simulink model "QuadrotorSim"  (R2019a)
settings: Solver=VariableStepAuto  StartTime=0.0  StopTime=inf  RelTol=1e-3
InitFcn:
  | close all; clear; clc;
  | mdl_quadrotor;
  | Para.d = 0.225;
  | Para.cT = 1.105e-5;
  | Para.cM = 1.779e-07;
  | Para.m = 1.4;
  | Para.Inertia = diag([0.0211, 0.0219, 0.0366]);
  | 
  | g = 9.8;
libraries: simulink x6, shared6dof x1, roblocks x1
settings Model: Creator=Administrator  LastModifiedBy=Cybaster
settings DataIOCC: ReturnWorkspaceOutputs=off
settings DebuggingCC: ArithmeticOperatorsInVariantConditions=warning

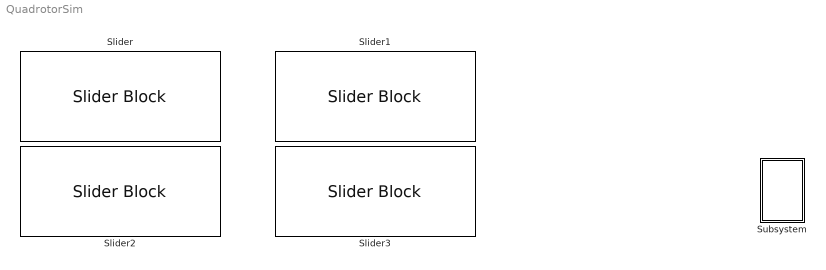
== system QuadrotorSim ==
  Slider : SliderBlock  ScaleMin=-2  ScaleMax=2
  Slider1 : SliderBlock  ScaleMin=-2  ScaleMax=2
  Slider2 : SliderBlock  ScaleMax=10
  Slider3 : SliderBlock  ScaleMin=-3.1400000000000001  ScaleMax=3.1400000000000001
  Subsystem : Subsystem

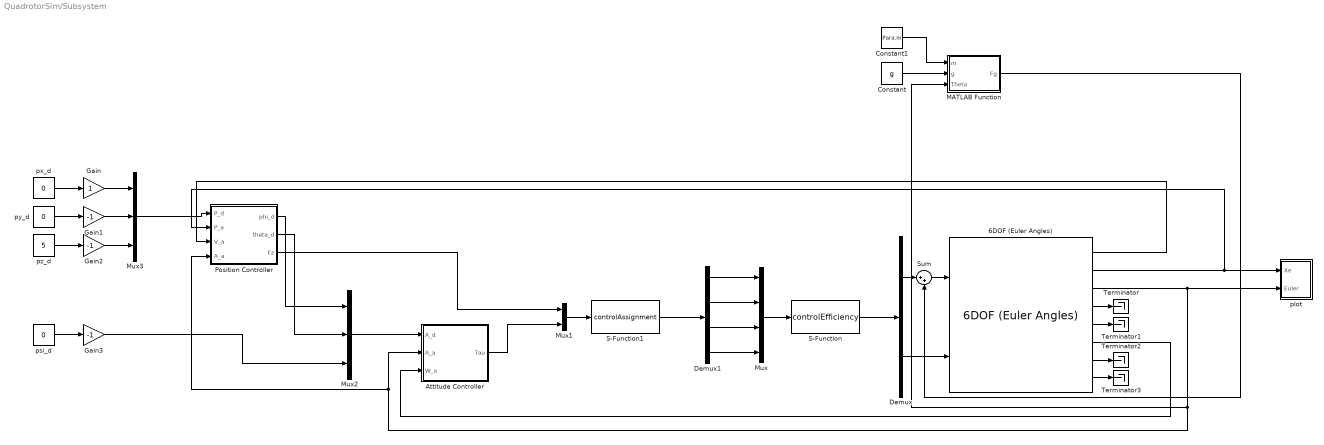
== system QuadrotorSim/Subsystem ==
  6DOF (Euler Angles) : shared6dof/6DOF (Euler Angles)  units=Metric (MKS)  mtype=Fixed  rep=Euler Angles  xme_0=[0.0 0.0 0.0]  Vm_0=[0.0 0.0 0.0]  eul_0=[0.0 0.0 0.0]  pm_0=[0.0 0.0 0.0]  mass_0=Para.m  mass_e=0.5  mass_f=2.0  inertia=Para.Inertia  inertia_e=eye(3)  inertia_f=2*eye(3)  k_quat=1.0  vre_flag=on  abi_flag=off  aMode=0  xme_statename=''  Vm_statename=''  eul_statename=''  quat_statename=''  pm_statename=''  mass_statename=''
      settings: SourceProductBaseCode=AE
  Attitude Controller : Subsystem
  Constant : Constant  Value=g
  Constant1 : Constant  Value=Para.m
  Demux : Demux  Outputs=2
  Demux1 : Demux
  Gain : Gain
  Gain1 : Gain  Gain=-1
  Gain2 : Gain  Gain=-1
  Gain3 : Gain  Gain=-1
  MATLAB Function : MATLAB Function  TreatAsAtomicUnit=on
  Mux : Mux
  Mux1 : Mux  Inputs=2
  Mux2 : Mux  Inputs=3
  Mux3 : Mux  Inputs=3
  Position Controller : Subsystem
  S-Function : S-Function  FunctionName=controlEfficiency  Parameters=Para  SFunctionDeploymentMode=off  EnableBusSupport=off
  S-Function1 : S-Function  FunctionName=controlAssignment  SFunctionDeploymentMode=off  EnableBusSupport=off
  Sum : Sum  Inputs=|++
  Terminator{,1..3} (4 alike) : Terminator
  plot : Subsystem
  psi_d : Constant  Value=0
  px_d : Constant  Value=0
  py_d : Constant  Value=0
  pz_d : Constant  Value=5
  wires:
  Demux1/1 -> Mux/1
  Demux/2 -> 6DOF (Euler Angles)/2
  Position Controller/2(theta_d) -> Mux2/2
  Mux1/1 -> S-Function1/1
  Mux3/1 -> Position Controller/1(P_d)
  6DOF (Euler Angles)/7 -> Terminator2/1
  Demux1/3 -> Mux/3
  Demux/1 -> Sum/1
  6DOF (Euler Angles)/3 -> MATLAB Function/3(Theta), Attitude Controller/2(A_a), Position Controller/4(A_a), plot/2(Euler)
  S-Function/1 -> Demux/1
  6DOF (Euler Angles)/8 -> Terminator3/1
  6DOF (Euler Angles)/4 -> Terminator/1
  6DOF (Euler Angles)/5 -> Terminator1/1
  6DOF (Euler Angles)/1 -> Position Controller/3(V_a)
  Gain2/1 -> Mux3/3
  Constant/1 -> MATLAB Function/2(g)
  Position Controller/1(phi_d) -> Mux2/1
  Gain1/1 -> Mux3/2
  Demux1/4 -> Mux/4
  6DOF (Euler Angles)/2 -> Position Controller/2(P_a), plot/1(Xe)
  Mux/1 -> S-Function/1
  Gain/1 -> Mux3/1
  py_d/1 -> Gain1/1
  Mux2/1 -> Attitude Controller/1(A_d)
  MATLAB Function/1(Fg) -> Sum/2
  px_d/1 -> Gain/1
  Attitude Controller/1(Tau) -> Mux1/2
  Position Controller/3(Fz) -> Mux1/1
  Sum/1 -> 6DOF (Euler Angles)/1
  Demux1/2 -> Mux/2
  6DOF (Euler Angles)/6 -> Attitude Controller/3(W_a)
  psi_d/1 -> Gain3/1
  S-Function1/1 -> Demux1/1
  Constant1/1 -> MATLAB Function/1(m)
  pz_d/1 -> Gain2/1
  Gain3/1 -> Mux2/3

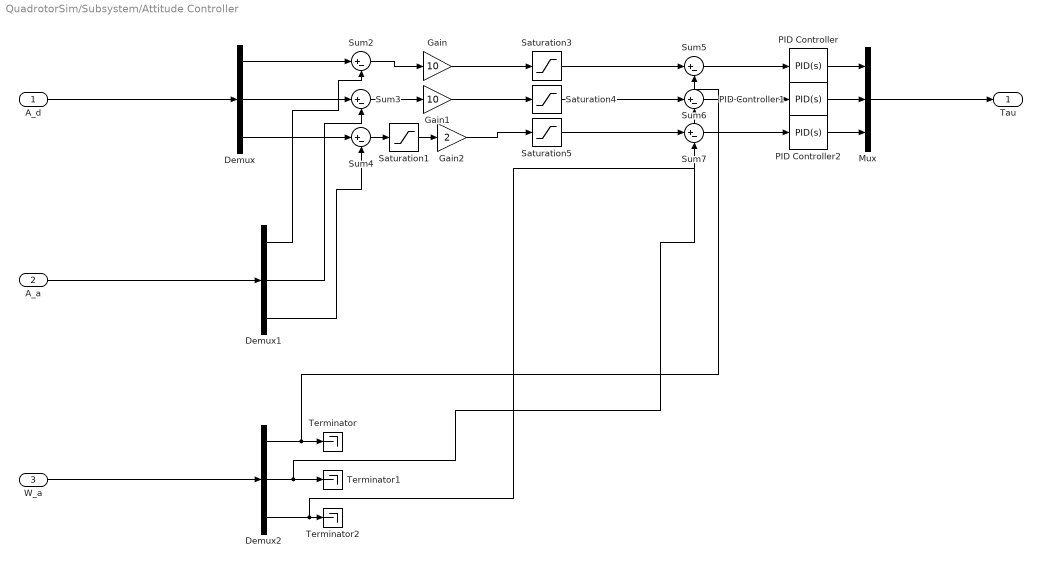
== system QuadrotorSim/Subsystem/Attitude Controller ==
  A_d : Inport
  A_a : Inport  Port=2
  W_a : Inport  Port=3
  Demux : Demux  Outputs=3
  Demux1 : Demux  Outputs=3
  Demux2 : Demux  Outputs=3
  Gain : Gain  Gain=10
  Gain1 : Gain  Gain=10
  Gain2 : Gain  Gain=2
  Mux : Mux  Inputs=3
  PID Controller : simulink/Continuous/PID Controller  Controller=PID  Form=Parallel  TimeDomain=Continuous-time  SampleTime=-1  IntegratorMethod=Forward Euler  FilterMethod=Forward Euler  ControllerParametersSource=internal  P=872359.79769725  I=16686702.0600055  D=-1838.38000156362  UseFilter=on  N=172.044274974478  TunerSelectOption=Transfer Function Based (PID Tuner App)  InitialConditionSource=internal  InitialConditionForIntegrator=0  InitialConditionForFilter=0  DifferentiatorICPrevScaledInput=0  ExternalReset=none  TrackingMode=off  Kt=1  LimitOutput=off  UpperSaturationLimit=inf  LowerSaturationLimit=-inf  LinearizeAsGain=on  AntiWindupMode=none  Kb=1  POutMin=[]  POutMax=[]  IOutMin=[]  IOutMax=[]  DOutMin=[]  DOutMax=[]  NOutMin=[]  NOutMax=[]  SumOutMin=[]  SumOutMax=[]  SaturationOutMin=[]  SaturationOutMax=[]  PParamMin=[]  PParamMax=[]  IParamMin=[]  IParamMax=[]  DParamMin=[]  DParamMax=[]  NParamMin=[]  NParamMax=[]  KbParamMin=[]  KbParamMax=[]  KtParamMin=[]  KtParamMax=[]  KbOutMin=[]  KbOutMax=[]  KtOutMin=[]  KtOutMax=[]  IntegratorOutMin=[]  IntegratorOutMax=[]  FilterOutMin=[]  FilterOutMax=[]  SumI1OutMin=[]  SumI1OutMax=[]  SumI2OutMin=[]  SumI2OutMax=[]  SumI3OutMin=[]  SumI3OutMax=[]  SumI4OutMin=[]  SumI4OutMax=[]  SumDOutMin=[]  SumDOutMax=[]  DifferentiatorOutMin=[]  DifferentiatorOutMax=[]  FilterDiffOutCoefMin=[]  FilterDiffOutCoefMax=[]  ReciprocalOutMin=[]  ReciprocalOutMax=[]  SumDenOutMin=[]  SumDenOutMax=[]  SumNumOutMin=[]  SumNumOutMax=[]  DivideOutMin=[]  DivideOutMax=[]  IntegratorContinuousStateAttributes=''  IntegratorStateMustResolveToSignalObject=off  IntegratorRTWStateStorageClass=Auto  FilterContinuousStateAttributes=''  FilterStateMustResolveToSignalObject=off  FilterRTWStateStorageClass=Auto  ParallelPVariant=InternalParameters  IdealPVariant=Disabled  IVariant=InternalParameters  DVariant=InternalParameters  IntegratorVariant=Continuous  SatVariant=Disabled  AWVariant=Passthrough  PCopyVariant=Disabled  TRVariant=Disabled  FdbkBlocksVariant=Forward  IdealPFdbkVariant=Disabled  SatFdbkVariant=Disabled  DerivativeFilterVariant=ContFilter  NVariant=InternalParameters  NCopyVariant=Disabled  FilterICVariant=InternalICsFilter  IntegratorICVariant=InternalICs  ExternalResetVariant=Disabled  TRSumVariant=Passthrough  SumFdbkVariant=Disabled  SumVariant=Sum_PID
  PID Controller1 : simulink/Continuous/PID Controller  Controller=PID  Form=Parallel  TimeDomain=Continuous-time  SampleTime=-1  IntegratorMethod=Forward Euler  FilterMethod=Forward Euler  ControllerParametersSource=internal  P=905409.552147454  I=17318885.4860674  D=-1908.02787827485  UseFilter=on  N=172.044274974478  TunerSelectOption=Transfer Function Based (PID Tuner App)  InitialConditionSource=internal  InitialConditionForIntegrator=0  InitialConditionForFilter=0  DifferentiatorICPrevScaledInput=0  ExternalReset=none  TrackingMode=off  Kt=1  LimitOutput=off  UpperSaturationLimit=inf  LowerSaturationLimit=-inf  LinearizeAsGain=on  AntiWindupMode=none  Kb=1  POutMin=[]  POutMax=[]  IOutMin=[]  IOutMax=[]  DOutMin=[]  DOutMax=[]  NOutMin=[]  NOutMax=[]  SumOutMin=[]  SumOutMax=[]  SaturationOutMin=[]  SaturationOutMax=[]  PParamMin=[]  PParamMax=[]  IParamMin=[]  IParamMax=[]  DParamMin=[]  DParamMax=[]  NParamMin=[]  NParamMax=[]  KbParamMin=[]  KbParamMax=[]  KtParamMin=[]  KtParamMax=[]  KbOutMin=[]  KbOutMax=[]  KtOutMin=[]  KtOutMax=[]  IntegratorOutMin=[]  IntegratorOutMax=[]  FilterOutMin=[]  FilterOutMax=[]  SumI1OutMin=[]  SumI1OutMax=[]  SumI2OutMin=[]  SumI2OutMax=[]  SumI3OutMin=[]  SumI3OutMax=[]  SumI4OutMin=[]  SumI4OutMax=[]  SumDOutMin=[]  SumDOutMax=[]  DifferentiatorOutMin=[]  DifferentiatorOutMax=[]  FilterDiffOutCoefMin=[]  FilterDiffOutCoefMax=[]  ReciprocalOutMin=[]  ReciprocalOutMax=[]  SumDenOutMin=[]  SumDenOutMax=[]  SumNumOutMin=[]  SumNumOutMax=[]  DivideOutMin=[]  DivideOutMax=[]  IntegratorContinuousStateAttributes=''  IntegratorStateMustResolveToSignalObject=off  IntegratorRTWStateStorageClass=Auto  FilterContinuousStateAttributes=''  FilterStateMustResolveToSignalObject=off  FilterRTWStateStorageClass=Auto  ParallelPVariant=InternalParameters  IdealPVariant=Disabled  IVariant=InternalParameters  DVariant=InternalParameters  IntegratorVariant=Continuous  SatVariant=Disabled  AWVariant=Passthrough  PCopyVariant=Disabled  TRVariant=Disabled  FdbkBlocksVariant=Forward  IdealPFdbkVariant=Disabled  SatFdbkVariant=Disabled  DerivativeFilterVariant=ContFilter  NVariant=InternalParameters  NCopyVariant=Disabled  FilterICVariant=InternalICsFilter  IntegratorICVariant=InternalICs  ExternalResetVariant=Disabled  TRSumVariant=Passthrough  SumFdbkVariant=Disabled  SumVariant=Sum_PID
  PID Controller2 : simulink/Continuous/PID Controller  Controller=PID  Form=Parallel  TimeDomain=Continuous-time  SampleTime=-1  IntegratorMethod=Forward Euler  FilterMethod=Forward Euler  ControllerParametersSource=internal  P=21140502.8119185  I=404380477.817044  D=-44550.7435063145  UseFilter=on  N=172.044274974478  TunerSelectOption=Transfer Function Based (PID Tuner App)  InitialConditionSource=internal  InitialConditionForIntegrator=0  InitialConditionForFilter=0  DifferentiatorICPrevScaledInput=0  ExternalReset=none  TrackingMode=off  Kt=1  LimitOutput=off  UpperSaturationLimit=inf  LowerSaturationLimit=-inf  LinearizeAsGain=on  AntiWindupMode=none  Kb=1  POutMin=[]  POutMax=[]  IOutMin=[]  IOutMax=[]  DOutMin=[]  DOutMax=[]  NOutMin=[]  NOutMax=[]  SumOutMin=[]  SumOutMax=[]  SaturationOutMin=[]  SaturationOutMax=[]  PParamMin=[]  PParamMax=[]  IParamMin=[]  IParamMax=[]  DParamMin=[]  DParamMax=[]  NParamMin=[]  NParamMax=[]  KbParamMin=[]  KbParamMax=[]  KtParamMin=[]  KtParamMax=[]  KbOutMin=[]  KbOutMax=[]  KtOutMin=[]  KtOutMax=[]  IntegratorOutMin=[]  IntegratorOutMax=[]  FilterOutMin=[]  FilterOutMax=[]  SumI1OutMin=[]  SumI1OutMax=[]  SumI2OutMin=[]  SumI2OutMax=[]  SumI3OutMin=[]  SumI3OutMax=[]  SumI4OutMin=[]  SumI4OutMax=[]  SumDOutMin=[]  SumDOutMax=[]  DifferentiatorOutMin=[]  DifferentiatorOutMax=[]  FilterDiffOutCoefMin=[]  FilterDiffOutCoefMax=[]  ReciprocalOutMin=[]  ReciprocalOutMax=[]  SumDenOutMin=[]  SumDenOutMax=[]  SumNumOutMin=[]  SumNumOutMax=[]  DivideOutMin=[]  DivideOutMax=[]  IntegratorContinuousStateAttributes=''  IntegratorStateMustResolveToSignalObject=off  IntegratorRTWStateStorageClass=Auto  FilterContinuousStateAttributes=''  FilterStateMustResolveToSignalObject=off  FilterRTWStateStorageClass=Auto  ParallelPVariant=InternalParameters  IdealPVariant=Disabled  IVariant=InternalParameters  DVariant=InternalParameters  IntegratorVariant=Continuous  SatVariant=Disabled  AWVariant=Passthrough  PCopyVariant=Disabled  TRVariant=Disabled  FdbkBlocksVariant=Forward  IdealPFdbkVariant=Disabled  SatFdbkVariant=Disabled  DerivativeFilterVariant=ContFilter  NVariant=InternalParameters  NCopyVariant=Disabled  FilterICVariant=InternalICsFilter  IntegratorICVariant=InternalICs  ExternalResetVariant=Disabled  TRSumVariant=Passthrough  SumFdbkVariant=Disabled  SumVariant=Sum_PID
  Saturation1 : Saturate  UpperLimit=0.05  LowerLimit=-0.05
  Saturation3 : Saturate  UpperLimit=0.2  LowerLimit=-0.2
  Saturation4 : Saturate  UpperLimit=0.2  LowerLimit=-0.2
  Saturation5 : Saturate  UpperLimit=0.2  LowerLimit=-0.2
  Sum{2..7} (6 alike) : Sum  Inputs=|+-
  Terminator : Terminator
  Terminator1 : Terminator
  Terminator2 : Terminator
  Tau : Outport
  wires:
  A_a/1 -> Demux1/1
  W_a/1 -> Demux2/1
  A_d/1 -> Demux/1
  Demux/1 -> Sum2/1
  Demux/2 -> Sum3/1
  Demux/3 -> Sum4/1
  Demux1/1 -> Sum2/2
  Demux1/2 -> Sum3/2
  Demux1/3 -> Sum4/2
  Mux/1 -> Tau/1
  Demux2/1 -> Sum5/2, Terminator/1
  Demux2/3 -> Sum7/2, Terminator2/1
  Demux2/2 -> Sum6/2, Terminator1/1
  Sum5/1 -> PID Controller/1
  Sum6/1 -> PID Controller1/1
  Sum7/1 -> PID Controller2/1
  Sum2/1 -> Gain/1
  Sum3/1 -> Gain1/1
  PID Controller2/1 -> Mux/3
  PID Controller1/1 -> Mux/2
  PID Controller/1 -> Mux/1
  Saturation3/1 -> Sum5/1
  Saturation4/1 -> Sum6/1
  Saturation5/1 -> Sum7/1
  Gain/1 -> Saturation3/1
  Gain1/1 -> Saturation4/1
  Gain2/1 -> Saturation5/1
  Sum4/1 -> Saturation1/1
  Saturation1/1 -> Gain2/1

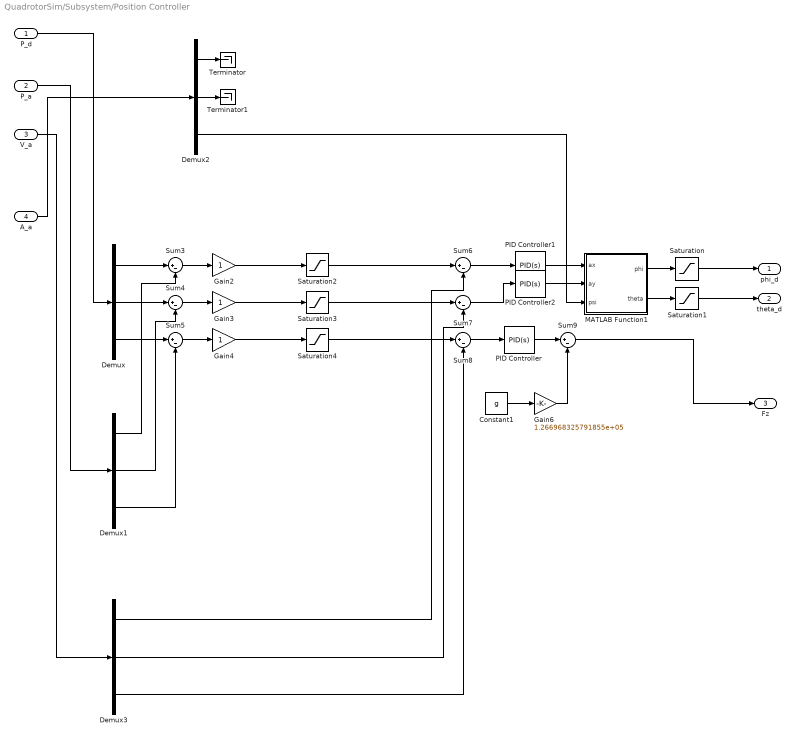
== system QuadrotorSim/Subsystem/Position Controller ==
  P_d : Inport
  P_a : Inport  Port=2
  V_a : Inport  Port=3
  A_a : Inport  Port=4
  Constant1 : Constant  Value=g
  Demux{,1..3} (4 alike) : Demux  Outputs=3
  Gain2 : Gain
  Gain3 : Gain
  Gain4 : Gain
  Gain6 : Gain  Gain=1.266968325791855e+05
  MATLAB Function1 : MATLAB Function  TreatAsAtomicUnit=on
  PID Controller : simulink/Continuous/PID Controller  Controller=PID  Form=Parallel  TimeDomain=Continuous-time  SampleTime=-1  IntegratorMethod=Forward Euler  FilterMethod=Forward Euler  ControllerParametersSource=internal  P=1301963.56478824  I=2490426.33050633  D=-27437.1169623964  UseFilter=on  N=17.2044274974478  TunerSelectOption=Transfer Function Based (PID Tuner App)  InitialConditionSource=internal  InitialConditionForIntegrator=0  InitialConditionForFilter=0  DifferentiatorICPrevScaledInput=0  ExternalReset=none  TrackingMode=off  Kt=1  LimitOutput=off  UpperSaturationLimit=inf  LowerSaturationLimit=-inf  LinearizeAsGain=on  AntiWindupMode=none  Kb=1  POutMin=[]  POutMax=[]  IOutMin=[]  IOutMax=[]  DOutMin=[]  DOutMax=[]  NOutMin=[]  NOutMax=[]  SumOutMin=[]  SumOutMax=[]  SaturationOutMin=[]  SaturationOutMax=[]  PParamMin=[]  PParamMax=[]  IParamMin=[]  IParamMax=[]  DParamMin=[]  DParamMax=[]  NParamMin=[]  NParamMax=[]  KbParamMin=[]  KbParamMax=[]  KtParamMin=[]  KtParamMax=[]  KbOutMin=[]  KbOutMax=[]  KtOutMin=[]  KtOutMax=[]  IntegratorOutMin=[]  IntegratorOutMax=[]  FilterOutMin=[]  FilterOutMax=[]  SumI1OutMin=[]  SumI1OutMax=[]  SumI2OutMin=[]  SumI2OutMax=[]  SumI3OutMin=[]  SumI3OutMax=[]  SumI4OutMin=[]  SumI4OutMax=[]  SumDOutMin=[]  SumDOutMax=[]  DifferentiatorOutMin=[]  DifferentiatorOutMax=[]  FilterDiffOutCoefMin=[]  FilterDiffOutCoefMax=[]  ReciprocalOutMin=[]  ReciprocalOutMax=[]  SumDenOutMin=[]  SumDenOutMax=[]  SumNumOutMin=[]  SumNumOutMax=[]  DivideOutMin=[]  DivideOutMax=[]  IntegratorContinuousStateAttributes=''  IntegratorStateMustResolveToSignalObject=off  IntegratorRTWStateStorageClass=Auto  FilterContinuousStateAttributes=''  FilterStateMustResolveToSignalObject=off  FilterRTWStateStorageClass=Auto  ParallelPVariant=InternalParameters  IdealPVariant=Disabled  IVariant=InternalParameters  DVariant=InternalParameters  IntegratorVariant=Continuous  SatVariant=Disabled  AWVariant=Passthrough  PCopyVariant=Disabled  TRVariant=Disabled  FdbkBlocksVariant=Forward  IdealPFdbkVariant=Disabled  SatFdbkVariant=Disabled  DerivativeFilterVariant=ContFilter  NVariant=InternalParameters  NCopyVariant=Disabled  FilterICVariant=InternalICsFilter  IntegratorICVariant=InternalICs  ExternalResetVariant=Disabled  TRSumVariant=Passthrough  SumFdbkVariant=Disabled  SumVariant=Sum_PID
  PID Controller1 : simulink/Continuous/PID Controller  Controller=PID  Form=Parallel  TimeDomain=Continuous-time  SampleTime=-1  IntegratorMethod=Forward Euler  FilterMethod=Forward Euler  ControllerParametersSource=internal  P=27.6032163785103  I=16.1035201553777  D=10.5128272922887  UseFilter=on  N=11428.279760416  TunerSelectOption=Transfer Function Based (PID Tuner App)  InitialConditionSource=internal  InitialConditionForIntegrator=0  InitialConditionForFilter=0  DifferentiatorICPrevScaledInput=0  ExternalReset=none  TrackingMode=off  Kt=1  LimitOutput=off  UpperSaturationLimit=inf  LowerSaturationLimit=-inf  LinearizeAsGain=on  AntiWindupMode=none  Kb=1  POutMin=[]  POutMax=[]  IOutMin=[]  IOutMax=[]  DOutMin=[]  DOutMax=[]  NOutMin=[]  NOutMax=[]  SumOutMin=[]  SumOutMax=[]  SaturationOutMin=[]  SaturationOutMax=[]  PParamMin=[]  PParamMax=[]  IParamMin=[]  IParamMax=[]  DParamMin=[]  DParamMax=[]  NParamMin=[]  NParamMax=[]  KbParamMin=[]  KbParamMax=[]  KtParamMin=[]  KtParamMax=[]  KbOutMin=[]  KbOutMax=[]  KtOutMin=[]  KtOutMax=[]  IntegratorOutMin=[]  IntegratorOutMax=[]  FilterOutMin=[]  FilterOutMax=[]  SumI1OutMin=[]  SumI1OutMax=[]  SumI2OutMin=[]  SumI2OutMax=[]  SumI3OutMin=[]  SumI3OutMax=[]  SumI4OutMin=[]  SumI4OutMax=[]  SumDOutMin=[]  SumDOutMax=[]  DifferentiatorOutMin=[]  DifferentiatorOutMax=[]  FilterDiffOutCoefMin=[]  FilterDiffOutCoefMax=[]  ReciprocalOutMin=[]  ReciprocalOutMax=[]  SumDenOutMin=[]  SumDenOutMax=[]  SumNumOutMin=[]  SumNumOutMax=[]  DivideOutMin=[]  DivideOutMax=[]  IntegratorContinuousStateAttributes=''  IntegratorStateMustResolveToSignalObject=off  IntegratorRTWStateStorageClass=Auto  FilterContinuousStateAttributes=''  FilterStateMustResolveToSignalObject=off  FilterRTWStateStorageClass=Auto  ParallelPVariant=InternalParameters  IdealPVariant=Disabled  IVariant=InternalParameters  DVariant=InternalParameters  IntegratorVariant=Continuous  SatVariant=Disabled  AWVariant=Passthrough  PCopyVariant=Disabled  TRVariant=Disabled  FdbkBlocksVariant=Forward  IdealPFdbkVariant=Disabled  SatFdbkVariant=Disabled  DerivativeFilterVariant=ContFilter  NVariant=InternalParameters  NCopyVariant=Disabled  FilterICVariant=InternalICsFilter  IntegratorICVariant=InternalICs  ExternalResetVariant=Disabled  TRSumVariant=Passthrough  SumFdbkVariant=Disabled  SumVariant=Sum_PID
  PID Controller2 : simulink/Continuous/PID Controller  Controller=PID  Form=Parallel  TimeDomain=Continuous-time  SampleTime=-1  IntegratorMethod=Forward Euler  FilterMethod=Forward Euler  ControllerParametersSource=internal  P=27.6039829287864  I=16.103967355358  D=10.513119236914  UseFilter=on  N=11428.279760416  TunerSelectOption=Transfer Function Based (PID Tuner App)  InitialConditionSource=internal  InitialConditionForIntegrator=0  InitialConditionForFilter=0  DifferentiatorICPrevScaledInput=0  ExternalReset=none  TrackingMode=off  Kt=1  LimitOutput=off  UpperSaturationLimit=inf  LowerSaturationLimit=-inf  LinearizeAsGain=on  AntiWindupMode=none  Kb=1  POutMin=[]  POutMax=[]  IOutMin=[]  IOutMax=[]  DOutMin=[]  DOutMax=[]  NOutMin=[]  NOutMax=[]  SumOutMin=[]  SumOutMax=[]  SaturationOutMin=[]  SaturationOutMax=[]  PParamMin=[]  PParamMax=[]  IParamMin=[]  IParamMax=[]  DParamMin=[]  DParamMax=[]  NParamMin=[]  NParamMax=[]  KbParamMin=[]  KbParamMax=[]  KtParamMin=[]  KtParamMax=[]  KbOutMin=[]  KbOutMax=[]  KtOutMin=[]  KtOutMax=[]  IntegratorOutMin=[]  IntegratorOutMax=[]  FilterOutMin=[]  FilterOutMax=[]  SumI1OutMin=[]  SumI1OutMax=[]  SumI2OutMin=[]  SumI2OutMax=[]  SumI3OutMin=[]  SumI3OutMax=[]  SumI4OutMin=[]  SumI4OutMax=[]  SumDOutMin=[]  SumDOutMax=[]  DifferentiatorOutMin=[]  DifferentiatorOutMax=[]  FilterDiffOutCoefMin=[]  FilterDiffOutCoefMax=[]  ReciprocalOutMin=[]  ReciprocalOutMax=[]  SumDenOutMin=[]  SumDenOutMax=[]  SumNumOutMin=[]  SumNumOutMax=[]  DivideOutMin=[]  DivideOutMax=[]  IntegratorContinuousStateAttributes=''  IntegratorStateMustResolveToSignalObject=off  IntegratorRTWStateStorageClass=Auto  FilterContinuousStateAttributes=''  FilterStateMustResolveToSignalObject=off  FilterRTWStateStorageClass=Auto  ParallelPVariant=InternalParameters  IdealPVariant=Disabled  IVariant=InternalParameters  DVariant=InternalParameters  IntegratorVariant=Continuous  SatVariant=Disabled  AWVariant=Passthrough  PCopyVariant=Disabled  TRVariant=Disabled  FdbkBlocksVariant=Forward  IdealPFdbkVariant=Disabled  SatFdbkVariant=Disabled  DerivativeFilterVariant=ContFilter  NVariant=InternalParameters  NCopyVariant=Disabled  FilterICVariant=InternalICsFilter  IntegratorICVariant=InternalICs  ExternalResetVariant=Disabled  TRSumVariant=Passthrough  SumFdbkVariant=Disabled  SumVariant=Sum_PID
  Saturation : Saturate  UpperLimit=0.15  LowerLimit=-0.15
  Saturation1 : Saturate  UpperLimit=0.15  LowerLimit=-0.15
  Saturation2 : Saturate  UpperLimit=0.1  LowerLimit=-0.1
  Saturation3 : Saturate  UpperLimit=0.1  LowerLimit=-0.1
  Saturation4 : Saturate  UpperLimit=0.1  LowerLimit=-0.1
  Sum{3..9} (7 alike) : Sum  Inputs=|+-
  Terminator : Terminator
  Terminator1 : Terminator
  phi_d : Outport
  theta_d : Outport  Port=2
  Fz : Outport  Port=3
  wires:
  P_a/1 -> Demux1/1
  P_d/1 -> Demux/1
  V_a/1 -> Demux3/1
  MATLAB Function1/1(phi) -> Saturation/1
  MATLAB Function1/2(theta) -> Saturation1/1
  Demux/1 -> Sum3/1
  Demux/2 -> Sum4/1
  Demux/3 -> Sum5/1
  Demux1/1 -> Sum3/2
  Demux1/2 -> Sum4/2
  Demux1/3 -> Sum5/2
  Sum3/1 -> Gain2/1
  Sum4/1 -> Gain3/1
  Sum5/1 -> Gain4/1
  Demux3/1 -> Sum6/2
  Demux3/2 -> Sum7/2
  Demux3/3 -> Sum8/2
  Sum8/1 -> PID Controller/1
  Sum9/1 -> Fz/1
  Constant1/1 -> Gain6/1
  Gain6/1 -> Sum9/2
  A_a/1 -> Demux2/1
  Demux2/1 -> Terminator/1
  Demux2/2 -> Terminator1/1
  Saturation/1 -> phi_d/1
  Saturation1/1 -> theta_d/1
  Sum6/1 -> PID Controller1/1
  PID Controller2/1 -> MATLAB Function1/2(ay)
  Sum7/1 -> PID Controller2/1
  PID Controller1/1 -> MATLAB Function1/1(ax)
  PID Controller/1 -> Sum9/1
  Gain2/1 -> Saturation2/1
  Saturation2/1 -> Sum6/1
  Gain4/1 -> Saturation4/1
  Gain3/1 -> Saturation3/1
  Saturation3/1 -> Sum7/1
  Saturation4/1 -> Sum8/1
  Demux2/3 -> MATLAB Function1/3(psi)

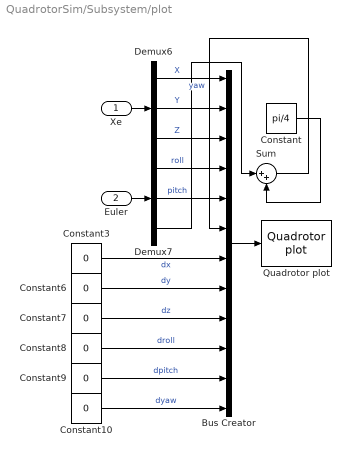
== system QuadrotorSim/Subsystem/plot ==
  Xe : Inport
  Euler : Inport  Port=2
  Bus Creator : BusCreator  Inputs=12
  Constant : Constant  Value=pi/4
  Constant{3,6..10} (6 alike) : Constant  Value=0
  Demux6 : Demux  Outputs=3
  Demux7 : Demux  Outputs=3
  Quadrotor plot : roblocks/Vehicles/Quadrotor plot  quad=quadrotor  xydim=2  zdim=10
  Sum : Sum  Inputs=|++
  wires:
  Constant10/1 -> Bus Creator/12  "dyaw"
  Bus Creator/1 -> Quadrotor plot/1
  Constant7/1 -> Bus Creator/9  "dz"
  Demux6/1 -> Bus Creator/1  "X"
  Constant8/1 -> Bus Creator/10  "droll"
  Constant9/1 -> Bus Creator/11  "dpitch"
  Demux7/2 -> Bus Creator/5  "pitch"
  Constant6/1 -> Bus Creator/8  "dy"
  Constant3/1 -> Bus Creator/7  "dx"
  Demux6/2 -> Bus Creator/2  "Y"
  Demux6/3 -> Bus Creator/3  "Z"
  Euler/1 -> Demux7/1
  Xe/1 -> Demux6/1
  Demux7/1 -> Bus Creator/4  "roll"
  Demux7/3 -> Sum/1
  Constant/1 -> Sum/2
  Sum/1 -> Bus Creator/6  "yaw"

== matlab function QuadrotorSim/Subsystem/MATLAB Function ==
  data: m input; g input; Fg output; Theta input
function Fg = fcn(m, g, Theta)
phi = Theta(1);
theta = Theta(2);
psi = Theta(3);

R = rotZ(psi) * rotY(theta) * rotX(phi);
G = [0; 0; g] * m;

Fg = R' * G;

== matlab function QuadrotorSim/Subsystem/Position Controller/MATLAB Function1 ==
  data: ax input; phi output; ay input; theta output; psi input
function [phi, theta] = fcn(ax, ay, psi)

g = 9.8;
A_hr = [ax; ay];
% A_psi = [cos(psi), sin(psi);
%     sin(psi), -cos(psi)];
A_psi = [sin(psi), cos(psi);
    -cos(psi), sin(psi)];

Theta = - 1/g * pinv(A_psi) * A_hr;

phi = Theta(1);
theta = Theta(2);
